simulink model "Motor_H_bridge"  (R2022b)
settings: Solver=FixedStepDiscrete  StartTime=0.0  StopTime=20  FixedStep=1e-6  RelTol=1e-3
libraries: spsDiodeLib x12, spsMosfetLib x8, spsCurrentMeasurementLib x2, spsDCMachineLib x2, spsDCVoltageSourceLib x2, spsParallelRLCBranchLib x2, spsThreePhaseSourceLib x2, spsVoltageMeasurementLib x2, spspowerguiLib x2
settings Model: Creator=smlmc  LastModifiedBy=smlmc

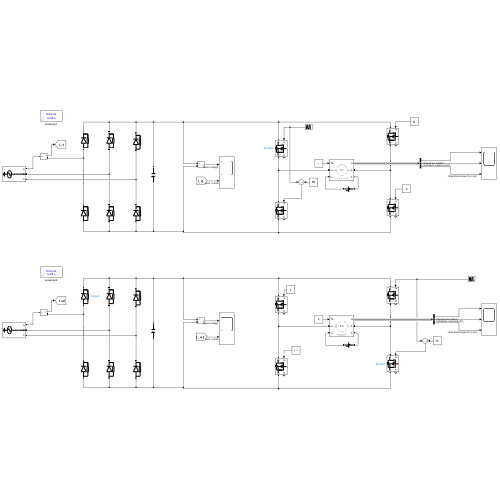
[thumbnail: Simulink's stored preview of the top-level diagram]
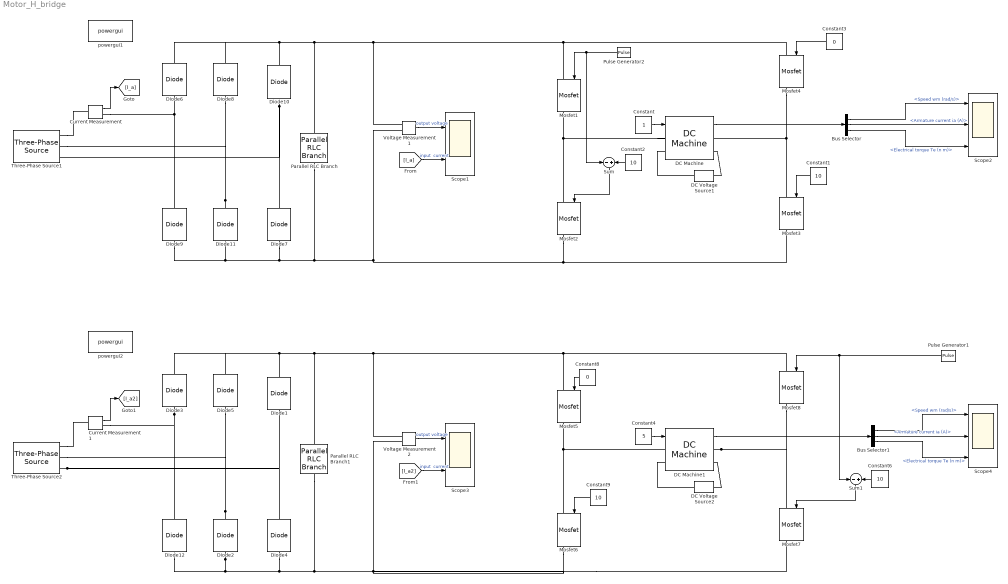
== system Motor_H_bridge ==
  Bus Selector : BusSelector  OutputSignals=Speed wm (rad/s),Armature current ia (A),Electrical torque Te (n m)
  Bus Selector1 : BusSelector  OutputSignals=Speed wm (rad/s),Armature current ia (A),Electrical torque Te (n m)
  Constant : Constant
  Constant{1..2,6,9} (4 alike) : Constant  Value=10
  Constant3 : Constant  Value=0
  Constant4 : Constant  Value=5
  Constant8 : Constant  Value=0
  Current Measurement : spsCurrentMeasurementLib/Current Measurement  PhasorSimulation=off  OutputType=Complex  PSBequivalent=0
  Current Measurement1 : spsCurrentMeasurementLib/Current Measurement  PhasorSimulation=off  OutputType=Complex  PSBequivalent=0
  DC Machine : spsDCMachineLib/DC Machine  PresetModel=No  MechanicalLoad=Torque TL  FieldType=Wound  ShowDetailedParameters=on  MeasurementBus=off  RLa="[ 0.8  0.0125]"  RLf="[210  23]"  Laf=1.3  MachineConstant=Torque constant (N.m/A)  Ke=1.8  Kt=1.8  J=0.2  Bm=0  Tf=0  w0=0  Ifinit=1.04761904756944  TsPowergui=0  TsBlock=-1
  DC Machine1 : spsDCMachineLib/DC Machine  PresetModel=No  MechanicalLoad=Torque TL  FieldType=Wound  ShowDetailedParameters=on  MeasurementBus=off  RLa="[ 0.8  0.0125]"  RLf="[210  23]"  Laf=1.3  MachineConstant=Torque constant (N.m/A)  Ke=1.8  Kt=1.8  J=0.4  Bm=0  Tf=0  w0=0  Ifinit=1.04761904756944  TsPowergui=0  TsBlock=-1
  DC Voltage Source1 : spsDCVoltageSourceLib/DC Voltage Source  Amplitude=220  Measurements=None
  DC Voltage Source2 : spsDCVoltageSourceLib/DC Voltage Source  Amplitude=220  Measurements=None
  Diode{1..12} (12 alike) : spsDiodeLib/Diode  Ron=0.00001  Lon=0  Vf=0.001  IC=0  UseSnubber=0  Rs=500  Cs=250e-9  Measurements=off
  Mosfet{1..8} (8 alike) : spsMosfetLib/Mosfet  Ron=0.1  Lon=0  Rd=0.01  Vfd=0  IC=0  Rs=1e5  Cs=inf  Measurements=on
  Parallel RLC Branch : spsParallelRLCBranchLib/Parallel RLC Branch  LConnTagsString=a  RConnTagsString=__new0  BranchType=C  Resistance=1  Inductance=1e-3  SetiL0=off  InitialCurrent=0  Capacitance=470e-6  Setx0=off  InitialVoltage=0  Measurements=None
  Parallel RLC Branch1 : spsParallelRLCBranchLib/Parallel RLC Branch  LConnTagsString=a  RConnTagsString=__new0  BranchType=C  Resistance=1  Inductance=1e-3  SetiL0=off  InitialCurrent=0  Capacitance=470e-6  Setx0=off  InitialVoltage=0  Measurements=None
  Pulse Generator1 : DiscretePulseGenerator  PulseType=Time based  Amplitude=10  Period=1e-4  PulseWidth=90  PhaseDelay=1e-6
  Pulse Generator2 : DiscretePulseGenerator  PulseType=Time based  Amplitude=10  Period=1e-4  PulseWidth=99  PhaseDelay=1e-6
  Scope1 : Scope  NumInputPorts=2
  Scope2 : Scope  NumInputPorts=3
  Scope3 : Scope  NumInputPorts=2
  Scope4 : Scope  NumInputPorts=3
  Sum : Sum  Inputs=-|+
  Sum1 : Sum  Inputs=-|+
  Three-Phase Source1 : spsThreePhaseSourceLib/Three-Phase Source  InternalConnection=Yg  VoltagePhases=off  Voltage=150  PhaseAngle=0  Voltage_phases=[25e3 25e3 25e3]/sqrt(3)  PhaseAngles_phases=[0 -120 +120]  Frequency=50  NonIdealSource=off  SpecifyImpedance=off  Resistance=0  Inductance=0.0001  ShortCircuitLevel=100e6  BaseVoltage=230*sqrt(3)  XRratio=7  BusType=swing  Pref=10e3  Qref=0  Prefabc=[10e3, 10e3, 10e3]  Qrefabc=[0, 0, 0]  Qmin=-inf  Qmax=inf
  Three-Phase Source2 : spsThreePhaseSourceLib/Three-Phase Source  InternalConnection=Yg  VoltagePhases=off  Voltage=80  PhaseAngle=0  Voltage_phases=[25e3 25e3 25e3]/sqrt(3)  PhaseAngles_phases=[0 -120 +120]  Frequency=50  NonIdealSource=off  SpecifyImpedance=off  Resistance=0  Inductance=0.0001  ShortCircuitLevel=100e6  BaseVoltage=230*sqrt(3)  XRratio=7  BusType=swing  Pref=10e3  Qref=0  Prefabc=[10e3, 10e3, 10e3]  Qrefabc=[0, 0, 0]  Qmin=-inf  Qmax=inf
  Voltage Measurement1 : spsVoltageMeasurementLib/Voltage Measurement  PhasorSimulation=off  OutputType=Complex  PSBequivalent=0
  Voltage Measurement2 : spsVoltageMeasurementLib/Voltage Measurement  PhasorSimulation=off  OutputType=Complex  PSBequivalent=0
  powergui1 : spspowerguiLib/powergui  Priority=1  SimulationMode=Discrete  SampleTime=1e-6  frequency=60  Iterations=50  frequencyindice=0  Pbase=100e6  ErrMax=1e-4  UnitsV=kV  UnitsW=MW  buscounter=0  FunctionMessages=off  echomessages=off  EnableUseOfTLC=off  CurrentSourceSwitches=off  DisableSnubberDevices=off  DisableRonSwitches=off  DisableVfSwitches=off  DisplayEquations=off  AutomaticDiscreteSolvers=off  SolverType=Tustin/Backward Euler (TBE)  Interpol=off  ExternalGateDelay=off  methode=off  Ts=100  x0status=blocks  SPID=on  SwTol=0  HookPort=off  NonlinearTolerance=1e-4  nMaxIteration=100  ContinueOnMaxIteration=off  RestoreLinks=warning  ResistiveCurrentMeasurement=off  Frange=[0:2:500]  Ylog=off  Xlog=on  ShowGrid=off  save=off  variable=ZData  structure=0  ZoomFFT=off  StartTime=0.0  cycles=1  DisplayStyle=1  fundamental=60  FreqAxis=off  MaxFrequency=1000  frequencyindicesteady=1  RmsSteady=1  display=off
  powergui2 : spspowerguiLib/powergui  Priority=1  SimulationMode=Discrete  SampleTime=1e-6  frequency=60  Iterations=50  frequencyindice=0  Pbase=100e6  ErrMax=1e-4  UnitsV=kV  UnitsW=MW  buscounter=0  FunctionMessages=off  echomessages=off  EnableUseOfTLC=off  CurrentSourceSwitches=off  DisableSnubberDevices=off  DisableRonSwitches=off  DisableVfSwitches=off  DisplayEquations=off  AutomaticDiscreteSolvers=off  SolverType=Tustin/Backward Euler (TBE)  Interpol=off  ExternalGateDelay=off  methode=off  Ts=100  x0status=blocks  SPID=on  SwTol=0  HookPort=off  NonlinearTolerance=1e-4  nMaxIteration=100  ContinueOnMaxIteration=off  RestoreLinks=warning  ResistiveCurrentMeasurement=off  Frange=[0:2:500]  Ylog=off  Xlog=on  ShowGrid=off  save=off  variable=ZData  structure=0  ZoomFFT=off  StartTime=0.0  cycles=1  DisplayStyle=1  fundamental=60  FreqAxis=off  MaxFrequency=1000  frequencyindicesteady=1  RmsSteady=1  display=off
  wires:
  Current Measurement/1 -> [I_a]
  Voltage Measurement1/1 -> Scope1/1  "output voltage"
  [I_a] -> Scope1/2  "input  current"
  Constant/1 -> DC Machine/1
  Constant2/1 -> Sum/2
  Bus Selector/3 -> Scope2/3  "<Electrical torque Te (n m)>"
  Bus Selector/2 -> Scope2/2  "<Armature current ia (A)>"
  Bus Selector/1 -> Scope2/1  "<Speed wm (rad/s)>"
  DC Machine/1 -> Bus Selector/1
  Pulse Generator2/1 -> Mosfet1/1, Sum/1
  Constant1/1 -> Mosfet3/1
  Sum/1 -> Mosfet2/1
  Constant3/1 -> Mosfet4/1
  Bus Selector1/2 -> Scope4/2  "<Armature current ia (A)>"
  Bus Selector1/3 -> Scope4/3  "<Electrical torque Te (n m)>"
  Sum1/1 -> Mosfet7/1
  DC Machine1/1 -> Bus Selector1/1
  Current Measurement1/1 -> [I_a2]
  [I_a2] -> Scope3/2  "input  current"
  Voltage Measurement2/1 -> Scope3/1  "output voltage"
  Bus Selector1/1 -> Scope4/1  "<Speed wm (rad/s)>"
  Constant4/1 -> DC Machine1/1
  Pulse Generator1/1 -> Sum1/1, Mosfet8/1
  Constant6/1 -> Sum1/2
  Constant9/1 -> Mosfet6/1
  Constant8/1 -> Mosfet5/1
  connections:
  Diode11/RConn1 -- Diode8/LConn1 -- Three-Phase Source1/RConn2
  Mosfet2/RConn1 -- Mosfet3/RConn1 -- Diode7/LConn1 -- Diode9/LConn1 -- Diode11/LConn1 -- Parallel RLC Branch/RConn1 -- Voltage Measurement1/LConn2
  Diode10/LConn1 -- Diode7/RConn1 -- Three-Phase Source1/RConn3
  Diode9/RConn1 -- Current Measurement/RConn1 -- Diode6/LConn1
  Three-Phase Source1/RConn1 -- Current Measurement/LConn1
  DC Voltage Source1/RConn1 -- DC Machine/LConn2
  DC Voltage Source1/LConn1 -- DC Machine/RConn2
  DC Machine/LConn1 -- Mosfet1/RConn1 -- Mosfet2/LConn1
  Mosfet3/LConn1 -- Mosfet4/RConn1 -- DC Machine/RConn1
  Mosfet4/LConn1 -- Voltage Measurement1/LConn1 -- Parallel RLC Branch/LConn1 -- Diode10/RConn1 -- Diode8/RConn1 -- Diode6/RConn1 -- Mosfet1/LConn1
  Diode2/LConn1 -- Diode12/LConn1 -- Mosfet7/RConn1 -- Mosfet6/RConn1 -- Voltage Measurement2/LConn2 -- Parallel RLC Branch1/RConn1 -- Diode4/LConn1
  Mosfet8/LConn1 -- Mosfet5/LConn1 -- Voltage Measurement2/LConn1 -- Parallel RLC Branch1/LConn1 -- Diode1/RConn1 -- Diode5/RConn1 -- Diode3/RConn1
  Three-Phase Source2/RConn3 -- Diode4/RConn1 -- Diode1/LConn1
  Diode3/LConn1 -- Diode12/RConn1 -- Current Measurement1/RConn1
  DC Machine1/LConn1 -- Mosfet5/RConn1 -- Mosfet6/LConn1
  DC Machine1/RConn1 -- Mosfet8/RConn1 -- Mosfet7/LConn1
  Diode2/RConn1 -- Diode5/LConn1 -- Three-Phase Source2/RConn2
  DC Voltage Source2/LConn1 -- DC Machine1/RConn2
  DC Voltage Source2/RConn1 -- DC Machine1/LConn2
  Three-Phase Source2/RConn1 -- Current Measurement1/LConn1
